simulink model "pmsm_pid_ctl"  (R2023a)
settings: configuration reference "config" (kept outside this file)
model workspace (MATLAB code in the model file + MAT data in the model file):
  cmdLim = Simulink.Parameter
  cmdLim.Value = 15
  cmdLim.Description = 'Limit for controlling the maximum surface command angle.'
  cmdLim.Min = 0
  cmdLim.Max = 90
  cmdLim.DocUnits = 'deg'
  dispGain = Simulink.Parameter
  dispGain.Value = 0.75
  dispGain.Description = 'Gain applied to the displacement error.'
  dispGain.Min = 0
  dispGain.Max = []
  dispGain.DocUnits = 'deg/sec/deg'
  dispLim = Simulink.Parameter
  dispLim.Value = 30
  dispLim.Description = 'Limit for controlling the maximum commanded angle.'
  dispLim.Min = 0
  dispLim.Max = 180
  dispLim.DocUnits = 'deg'
  intGain = Simulink.Parameter
  intGain.Value = 0.5
  intGain.Description = 'Gain applied to the integral error.'
  intGain.Min = 0
  intGain.Max = []
  intGain.DocUnits = 'deg/sec/deg/sec'
  intLim = Simulink.Parameter
  intLim.Value = 5
  intLim.Description = 'Limit for controlling the maximum commanded angle.'
  intLim.Min = 0
  intLim.Max = 90
  intLim.DocUnits = 'deg'
  rateGain = Simulink.Parameter
  rateGain.Value = 2
  rateGain.Description = 'Gain applied to the rate error.'
  rateGain.Min = 0
  rateGain.Max = []
  rateGain.DocUnits = 'deg/deg/sec'
  rateLim = Simulink.Parameter
  rateLim.Value = 6
  rateLim.Description = 'Limit for controlling the maximum commanded angle.'
  rateLim.Min = 0
  rateLim.Max = 180
  rateLim.DocUnits = 'deg/sec'
  hdgGain = Simulink.Parameter
  hdgGain.Value = 0.015
  enc_line = Simulink.Parameter
  enc_line.Value = 4000
  enc_line.Description = '编码器分辨率 '
  enc_line.DataType = 'uint32'
  enc_line.Complexity = 'real'
  enc_line.Dimensions = [1 1]
  enc_line_init_pos = Simulink.Parameter
  enc_line_init_pos.Value = 0
  enc_line_init_pos.Description = '编码器初始位置'
  enc_line_init_pos.DataType = 'int64'
  enc_line_init_pos.Complexity = 'real'
  enc_line_init_pos.Dimensions = [1 1]
  enc_line_inv_p_n = Simulink.Parameter
  enc_line_inv_p_n.Value = 0.00025
  enc_line_inv_p_n.Description = '编码器分辨率 '
  enc_line_inv_p_n.DataType = 'single'
  enc_line_inv_p_n.Complexity = 'real'
  enc_line_inv_p_n.Dimensions = [1 1]
  iq_max = Simulink.Parameter
  iq_max.Value = 10
  iq_max.Description = 'iq 目标电流最大值 A'
  iq_max.DataType = 'single'
  iq_max.Complexity = 'real'
  iq_max.Dimensions = [1 1]
  tp = Simulink.Parameter
  tp.Value = 0.0001
  tp.Description = '位置环速度环执行周期'
  tp.DataType = 'double'
  tp.Complexity = 'real'
  tp.Dimensions = [1 1]
libraries: servo_hub_lib x1
settings Model: RequirementInfo={} %GIDa_fe9045fd_0412_4b6e_8206_617cc20e6fde  DataDictionary=model_config.sldd  ParameterArgumentNames=enc_line,enc_line_init_pos,enc_line_inv_p_n,iq_max  Creator=Administrator  LastModifiedBy=Administrator
settings ConfigSetRef: SourceName=config

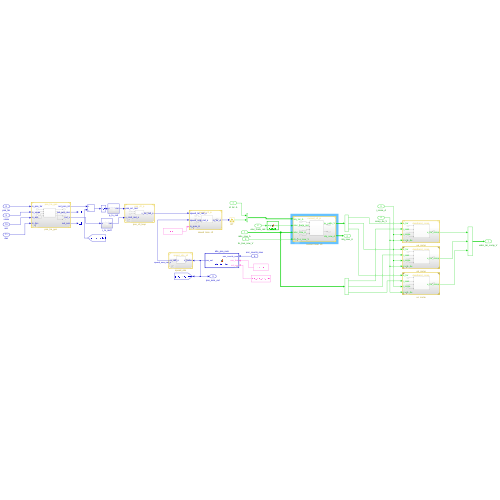
[thumbnail: Simulink's stored preview of the top-level diagram]
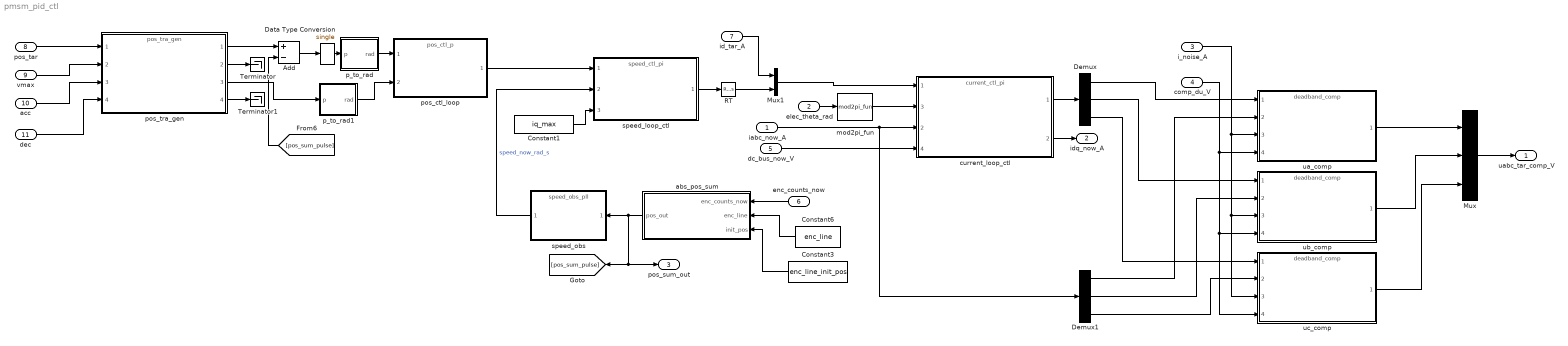
== system pmsm_pid_ctl ==
  iabc_now_A : Inport
  elec_theta_rad : Inport  Port=2
  i_noise_A : Inport  Port=3
  comp_du_V : Inport  Port=4
  dc_bus_now_V : Inport  Port=5
  enc_counts_now : Inport  Port=6  OutDataTypeStr=uint32
  id_tar_A : Inport  Port=7  OutDataTypeStr=single  SampleTime=5e-5
  pos_tar : Inport  Port=8
  vmax : Inport  Port=9
  acc : Inport  Port=10
  dec : Inport  Port=11
  Add : Sum  Inputs=+-
  Constant1 : Constant  Value=iq_max
  Constant3 : Constant  Value=enc_line_init_pos
  Constant6 : Constant  Value=enc_line  OutDataTypeStr=uint32
  Data Type Conversion : DataTypeConversion  OutDataTypeStr=single  SaturateOnIntegerOverflow=off  RndMeth=Floor
  Demux : Demux  Outputs=3
  Demux1 : Demux  Outputs=3
  Mux : Mux  Inputs=3
  Mux1 : Mux  Inputs=2
  RT : RateTransition  OutPortSampleTime=5e-05
  Terminator : Terminator
  Terminator1 : Terminator
  abs_pos_sum : MATLAB Function  TreatAsAtomicUnit=on  SystemSampleTime=tp
  current_loop_ctl : ModelReference  ModelNameDialog=current_ctl_pi.slx  UsingDefaultArgumentValue=0,0,0,0,0,0,0,0,0  SimulationMode=Normal  ModelReferenceVersion=2.139
      settings: PortSchema="{\"entries\":[{\"content\":{\"sides\":[{\"content\":{\"connectorIds\":[\"In1\",\"In3\",\"In2\",\"In4\"]},\"type\":\"ConnectorPlacement.EquallySpacedRectSide\",\"uuid\":\"465030fc-d4ed-4fad-a179-540c34c84031\"},{\"content\":{\"connectorIds\":[\"Out1\",\"Out2\"],\"side\":\"RIGHT\"},\"type\":\"ConnectorPlacement.EquallySpacedRectSide\",\"uuid\":\"fab44f7c-49ff-4c48-be02-a76080765122\"},{\"content\":{\"side\":\"TOP\"},\"type\":\"ConnectorPlacement.EquallySpacedRectSide\",\"uuid\":\"fa8fd0f2-cfd7-4f03-a40d-8124b2b913be\"}]},\"type\":\"ConnectorPlacement.EquallySpacedConnector\",\"uuid\":\"0e10ec8c-f9f2-4aaa-bb2e-fccf0700d204\"}],\"packageUris\":[\"http://schema.mathworks.com/mf0/Connector/R2020b\"],\"version\":\"1.0\"}"
  mod2pi_fun : servo_hub_lib/fast_math/mod2pi_fun  SystemSampleTime=-1  VariantActivationTime=update diagram  Latency=0  AutoFrameSizeCalculation=off
      settings: LibrarySourceBlock=|
      | simulink/User-Defined
      | Functions/MATLAB Function
  p_to_rad : Subsystem
  p_to_rad1 : Subsystem
  pos_ctl_loop : ModelReference  ModelNameDialog=pos_ctl_p.slx  UsingDefaultArgumentValue=0,0,0  SimulationMode=Normal  ModelReferenceVersion=2.45
  pos_tra_gen : ModelReference  ModelNameDialog=pos_tra_gen.slx  UsingDefaultArgumentValue=0  SimulationMode=Normal  ModelReferenceVersion=2.26
  speed_loop_ctl : ModelReference  ModelNameDialog=speed_ctl_pi.slx  UsingDefaultArgumentValue=0,0,0,0  SimulationMode=Normal  ModelReferenceVersion=1.174
  speed_obs : ModelReference  ModelNameDialog=speed_obs_pll.slx  UsingDefaultArgumentValue=0,0,0  SimulationMode=Normal  ModelReferenceVersion=2.254
  ua_comp : ModelReference  ModelNameDialog=deadband_comp.slx  SimulationMode=Normal  ModelReferenceVersion=1.149
  ub_comp : ModelReference  ModelNameDialog=deadband_comp.slx  SimulationMode=Normal  ModelReferenceVersion=1.149
  uc_comp : ModelReference  ModelNameDialog=deadband_comp.slx  SimulationMode=Normal  ModelReferenceVersion=1.149
  uabc_tar_comp_V : Outport
  idq_now_A : Outport  Port=2
  pos_sum_out : Outport  Port=3
  wires:
  current_loop_ctl/1 -> Demux/1
  elec_theta_rad/1 -> mod2pi_fun/1
  iabc_now_A/1 -> Demux1/1, current_loop_ctl/2
  Demux/1 -> ua_comp/1
  Demux1/1 -> ua_comp/2
  Demux/2 -> ub_comp/1
  Demux/3 -> uc_comp/1
  Demux1/2 -> ub_comp/2
  Demux1/3 -> uc_comp/2
  i_noise_A/1 -> uc_comp/3, ub_comp/3, ua_comp/3
  comp_du_V/1 -> uc_comp/4, ub_comp/4, ua_comp/4
  ua_comp/1 -> Mux/1
  ub_comp/1 -> Mux/2
  uc_comp/1 -> Mux/3
  Mux/1 -> uabc_tar_comp_V/1
  current_loop_ctl/2 -> idq_now_A/1
  mod2pi_fun/1 -> current_loop_ctl/3
  dc_bus_now_V/1 -> current_loop_ctl/4
  speed_obs/1 -> speed_loop_ctl/2  "speed_now_rad_s"
  pos_ctl_loop/1 -> speed_loop_ctl/1
  abs_pos_sum/1(pos_out) -> [pos_sum_pulse], pos_sum_out/1, speed_obs/1
  Constant1/1 -> speed_loop_ctl/3
  RT/1 -> Mux1/2
  id_tar_A/1 -> Mux1/1
  Constant3/1 -> abs_pos_sum/3(init_pos)
  Constant6/1 -> abs_pos_sum/2(enc_line)
  enc_counts_now/1 -> abs_pos_sum/1(enc_counts_now)
  Mux1/1 -> current_loop_ctl/1
  speed_loop_ctl/1 -> RT/1
  [pos_sum_pulse] -> Add/2
  pos_tra_gen/3 -> p_to_rad1/1(p)
  p_to_rad/1(rad) -> pos_ctl_loop/1
  Add/1 -> Data Type Conversion/1
  Data Type Conversion/1 -> p_to_rad/1(p)
  pos_tra_gen/1 -> Add/1
  pos_tra_gen/2 -> Terminator/1
  pos_tra_gen/4 -> Terminator1/1
  p_to_rad1/1(rad) -> pos_ctl_loop/2
  pos_tar/1 -> pos_tra_gen/1
  vmax/1 -> pos_tra_gen/2
  acc/1 -> pos_tra_gen/3
  dec/1 -> pos_tra_gen/4

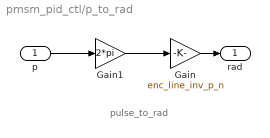
== system pmsm_pid_ctl/p_to_rad ==
  note: pulse_to_rad
  p : Inport
  Gain : Gain  Gain=enc_line_inv_p_n
  Gain1 : Gain  Gain=2*pi
  rad : Outport
  wires:
  p/1 -> Gain1/1
  Gain1/1 -> Gain/1
  Gain/1 -> rad/1

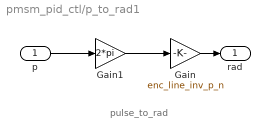
== system pmsm_pid_ctl/p_to_rad1 ==
  note: pulse_to_rad
  p : Inport
  Gain : Gain  Gain=enc_line_inv_p_n
  Gain1 : Gain  Gain=2*pi
  rad : Outport
  wires:
  Gain/1 -> rad/1
  Gain1/1 -> Gain/1
  p/1 -> Gain1/1

== matlab function pmsm_pid_ctl/abs_pos_sum ==
  data: enc_counts_now input; pos_out output; enc_line input; init_pos input
function pos_out = abs_pos_sum(enc_counts_now, enc_line, init_pos)

persistent pos_single_last;
if isempty(pos_single_last)
    pos_single_last = int64(0);  %位置单圈值上一次值
end

persistent pos_single_now;
if isempty(pos_single_now)
    pos_single_now = int64(0);  %位置单圈值
end

persistent pos_sum;
if isempty(pos_sum)
    pos_sum = int64(0);  %位置单圈值
end

persistent first_flag;
if isempty(first_flag)
    first_flag = uint8(0);  %初始化赋值
end

if first_flag == uint8(0)
    first_flag = uint8(1);
    pos_single_now = int64(enc_counts_now);
    pos_single_last = int64(enc_counts_now);
    pos_sum = init_pos;  %从当前值开始累加
end


add_pos = int64(0);

enc_line_half = int64(enc_line / uint32(2));
pos_single_now = int64(enc_counts_now);
add_enc_line = int64(enc_line);

add_pos = pos_single_now - pos_single_last;
pos_single_last = pos_single_now;  %记录上一次值


if add_pos > enc_line_half   %反向溢出
    add_pos = add_pos - add_enc_line;
elseif add_pos < -enc_line_half  %正向溢出
    add_pos = add_pos + add_enc_line;
end

pos_sum = pos_sum + add_pos;
pos_out = pos_sum;
